simulink library "cdsWfsPhase"  (Simulink 6.2)
settings Model: LastModifiedBy=rolf

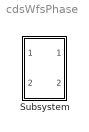
== system cdsWfsPhase ==
  Subsystem : Subsystem

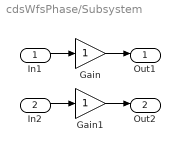
== system cdsWfsPhase/Subsystem ==
  In1 : Inport  Port=1  LatchInput=off
  In2 : Inport  Port=2  LatchInput=off
  Gain : Gain
  Gain1 : Gain
  Out1 : Outport
  Out2 : Outport  Port=2
  wires:
  In1/1 -> Gain/1
  Gain/1 -> Out1/1
  In2/1 -> Gain1/1
  Gain1/1 -> Out2/1
